simulink model "xEMU_SimulationModel3_rule1"  (R2017b)
settings: Solver=ode4  StartTime=0.0  StopTime=8192  FixedStep=0.01  RelTol=1e-3
undefined symbols (not defined in the file): a1, a2, a3, a4, ACO, BAT, Battery, DCT, DRT, EMS, ENV, Fahrzyklus_VS_modell, height_BAT, leistung, lib_bat, Maximum, Maximum_position, Num_cells, P_FC_max_long, P_FC_min_long, P_FC_step_max, Pbat_charge_max, Pbat_discharge_max, Pfc_max, Pfc_min, SOC_tar, time_peaks, TRM, velocity_peaks
libraries: simulink x5
(part 2 of 15)

== system xEMU_SimulationModel3_rule1/Fuel Cell System (FCS)/FC_controller  ==
  p_demand_ext : Inport
  V_dcLink : Inport  Port=2
  FC_state_BUS : Inport  Port=3
  V_FCS : Inport  Port=4
  p_fc_act : Inport  Port=5
  Add : Sum
  Bus Creator : BusCreator  Inputs=3
  Bus Creator1 : BusCreator  Inputs=5
  Constant : Constant  Value=42
  Constant1 : Constant  Value=P_FC_max_long
  Constant2 : Constant  Value=P_FC_step_max
  Constant4 : Constant  Value=P_FC_min_long
  Max : MinMax  Function=max  Inputs=2
  Min : MinMax  Inputs=2
  Product1 : Product  Inputs=*/
  Subtract : Sum  Inputs=+-
  Terminator : Terminator
  FCS_BUS : Outport
  i_demand : Outport  Port=2
  wires:
  Bus Creator1/1 -> Bus Creator/1
  FC_state_BUS/1 -> Bus Creator/2
  Constant/1 -> Bus Creator/3  "FCS_state"
  Add/1 -> Min/1
  Max/1 -> Bus Creator1/4  "P_FC_min"
  Min/1 -> Bus Creator1/2  "P_FC_max"
  Subtract/1 -> Max/1
  p_fc_act/1 -> Add/1, Subtract/1, Bus Creator1/1  "P_fc"
  Constant2/1 -> Add/2, Subtract/2
  Bus Creator/1 -> FCS_BUS/1
  V_dcLink/1 -> Terminator/1
  V_FCS/1 -> Product1/2
  Product1/1 -> i_demand/1
  Constant1/1 -> Min/2, Bus Creator1/3  "P_FC_max_long"
  Constant4/1 -> Max/2, Bus Creator1/5  "P_FC_min_long"
  p_demand_ext/1 -> Product1/1

== system xEMU_SimulationModel3_rule1/Fuel Cell System (FCS)/FC_system ==
  "P_fc " : Inport
  i_demand_dcdc_fc : Inport  Port=2
  1-D Lookup Table : Lookup_n-D  NumberOfTableDimensions=1  BreakpointsForDimension1=[0 10 20 50 126 241 270]  Table=[583 567 551 525 490 456 450]  InternalRulePriority=Speed  RndMeth=Simplest  InputSameDT=on
  Bus Creator : BusCreator  Inputs=2
  FaradayConstant : Constant  Commented=on  Value=96485
  FaradayConstant1 : Constant  Value=100
  MATLAB Function : MATLAB Function  TreatAsAtomicUnit=on
  NumCells : Constant  Commented=on  Value=Num_cells
  Product1 : Product  Commented=on  Inputs=/**
  Saturation : Saturate  UpperLimit=250  LowerLimit=0
  Scope : Scope
  Scope1 : Scope
  FCS_state_BUS : Outport
  V_FCS : Outport  Port=2
  i_act_fcs : Outport  Port=3
  wires:
  FaradayConstant1/1 -> Bus Creator/1  "H2_tankMass_kg"
  NumCells/1 -> Product1/3
  FaradayConstant/1 -> Product1/1
  Bus Creator/1 -> FCS_state_BUS/1
  1-D Lookup Table/1 -> Scope/1, V_FCS/1
  Saturation/1 -> Product1/2, i_act_fcs/1, 1-D Lookup Table/1
  i_demand_dcdc_fc/1 -> Scope1/1, Saturation/1
  MATLAB Function/1(H2_consumption_gramspersec) -> Bus Creator/2
  "P_fc "/1 -> MATLAB Function/1(xx)

== system xEMU_SimulationModel3_rule1/Scopes/Battery Scope ==
  Bus Selector : BusSelector  OutputSignals=V_bat,SOC,P_bat,I_bat
  Scope : Scope  NumInputPorts=3
  Scope1 : Scope
  Scope2 : Scope
  Scope6 : Scope
  wires:
  Bus Selector/1 -> Scope/1  "<V_bat>"
  [BAT_BUS] -> Bus Selector/1
  Bus Selector/2 -> Scope6/1  "<SOC>"
  [T_CellElement1] -> Scope1/1
  Bus Selector/3 -> Scope/3  "<P_bat>"
  Bus Selector/4 -> Scope2/1  "<I_bat>"

== system xEMU_SimulationModel3_rule1/Scopes/Energy Manager Scope ==
  Bus Selector1 : BusSelector  OutputSignals=P_acdc_Verlust,P_motor_mechanisch,P_motor_Verlust
  Bus Selector2 : BusSelector  OutputSignals=P_Klima
  Bus Selector3 : BusSelector  OutputSignals=P_bat
  Bus Selector4 : BusSelector  OutputSignals=signal1.P_fc
  Bus Selector5 : BusSelector  OutputSignals=P_dcdc_Verlust,P_dcLinkTractionLoad
  Divide : Product  Inputs=*/
  Integrator : Integrator
  Integrator1 : Integrator
  Leistung : Scope
  Leistung1 : Scope
  Leistung_verteilung : Scope
  Mux : Mux  Inputs=6
  Mux1 : Mux  Inputs=3
  wires:
  [DRT_BUS] -> Bus Selector1/1
  [DCT_BUS] -> Bus Selector5/1
  Mux/1 -> Leistung/1
  Bus Selector1/1 -> Mux/2  "<P_acdc_Verlust>"
  Bus Selector5/1 -> Integrator/1, Mux/5  "<P_dcdc_Verlust>"
  Bus Selector1/2 -> Mux/3  "<P_motor_mechanisch>"
  Bus Selector1/3 -> Mux/4  "<P_motor_Verlust>"
  [ACO_BUS] -> Bus Selector2/1
  Bus Selector2/1 -> Mux/6  "<P_Klima>"
  [APU_BUS] -> Mux/1
  [BAT_BUS] -> Bus Selector3/1
  Bus Selector3/1 -> Mux1/2  "<P_bat>"
  [FCS_BUS] -> Bus Selector4/1
  Bus Selector4/1 -> Mux1/3  "<P_fc>"
  Bus Selector5/2 -> Integrator1/1, Mux1/1  "<P_dcLinkTractionLoad>"
  Mux1/1 -> Leistung_verteilung/1
  Integrator/1 -> Divide/1
  Integrator1/1 -> Divide/2
  Divide/1 -> Leistung1/1

== system xEMU_SimulationModel3_rule1/Scopes/Fuel cell Scope  ==
  Bus Selector4 : BusSelector  OutputSignals=signal2.H2_tankMass_kg,signal2.H2_consumption_gramspersec
  Integrator : Integrator
  Scope : Scope  NumInputPorts=3
  wires:
  [FCS_BUS] -> Bus Selector4/1
  Bus Selector4/2 -> Scope/2, Integrator/1  "<H2_consumption_gramspersec>"
  Integrator/1 -> Scope/3  "Gesamtverbrauch_g"

== system xEMU_SimulationModel3_rule1/Scopes/Train Dynamics&Environment Scope ==
  Bus Selector1 : BusSelector  OutputSignals=v_drivingCycle_m/s,Steigung%
  Bus Selector2 : BusSelector  OutputSignals=v_train_m/s
  Integrator1 : Integrator
  Mux : Mux  Inputs=2
  Scope : Scope
  Scope2 : Scope
  V : Scope
  tag scope: distance=global
  wires:
  Bus Selector2/1 -> Mux/1  "<v_train_m/s>"
  [TRM_BUS] -> Bus Selector2/1
  [ENV_BUS] -> Bus Selector1/1
  Bus Selector1/1 -> Integrator1/1, Mux/2  "<v_drivingCycle_m/s>"
  Mux/1 -> V/1  "V_soll_VS_V_ist"
  Bus Selector1/2 -> Scope/1  "<Steigung%>"
  Integrator1/1 -> [distance], Scope2/1  "total distance"

== system xEMU_SimulationModel3_rule1/Train Dynamics (TRM)/Variant Subsystem ==
  v_drivingCycle_m/s : Inport
  h_drivingCycle_m : Inport  Port=2
  n_passengers_abs : Inport  Port=3
  adhesionCoefficient_abs : Inport  Port=4
  F_traction_N : Inport  Port=5
  v_s_model : Subsystem  VariantControl=Variant1
  v_t_model : Subsystem  VariantControl=Variant
  TRM_BUS : Outport
  F_tractionDemand_N : Outport  Port=2
  v_train_m/s : Outport  Port=3
  adhesionCoefficient : Outport  Port=4
  total_mass_kg : Outport  Port=5
  v_soll : Outport  Port=6

== system xEMU_SimulationModel3_rule1/Battery (BAT)_komplex/Subsystem/ActiveBalancing ==
  CellCurrents : Inport
  Demux : Demux  Outputs=1
  tag scope: ActBal1=global, BalancerBus=global
  wires:
  CellCurrents/1 -> Demux/1, [BalancerBus]
  Demux/1 -> [ActBal1]

== system xEMU_SimulationModel3_rule1/Battery (BAT)_komplex/Subsystem/CellCurrentMatrices ==
  Component0 : Subsystem
  Component1 : Subsystem
  Mux : Mux  Inputs=2
  Components : Outport
  wires:
  Mux/1 -> Components/1
  Component0/3(Value) -> Mux/1
  Component1/3(Value) -> Mux/2

== system xEMU_SimulationModel3_rule1/Battery (BAT)_komplex/Subsystem/CellCurrents ==
  CellCurrents : Inport
  Demux : Demux  Outputs=2
  Terminator : Terminator
  tag scope: I_CellElement1=global
  wires:
  CellCurrents/1 -> Demux/1
  Demux/2 -> Terminator/1
  Demux/1 -> [I_CellElement1]

== system xEMU_SimulationModel3_rule1/Battery (BAT)_komplex/Subsystem/CellPowerValues ==
  CellPower : Inport
  Demux : Demux  Outputs=1
  Out1 : Outport
  tag scope: P_CellElement1=global
  wires:
  CellPower/1 -> Out1/1, Demux/1  "CellPower"
  Demux/1 -> [P_CellElement1]

== system xEMU_SimulationModel3_rule1/Battery (BAT)_komplex/Subsystem/CellVoltageMatrices ==
  Component0 : Subsystem
  Component1 : Subsystem
  Mux : Mux  Inputs=2
  Components : Outport
  wires:
  Mux/1 -> Components/1
  Component0/3(Value) -> Mux/1
  Component1/3(Value) -> Mux/2

== system xEMU_SimulationModel3_rule1/Battery (BAT)_komplex/Subsystem/ElectricalCircuit ==
  Cellelement_Elem1 : Subsystem
  Out1 : Outport
  wires:
  Cellelement_Elem1/1(Out1) -> Out1/1

== system xEMU_SimulationModel3_rule1/Battery (BAT)_komplex/Subsystem/MatrixAxC ==
  StateComponent0 : Subsystem
  StateComponent1 : Subsystem
  StateComponent10 : Subsystem
  StateComponent11 : Subsystem
  StateComponent12 : Subsystem
  StateComponent13 : Subsystem
  StateComponent14 : Subsystem
  StateComponent15 : Subsystem
  StateComponent16 : Subsystem
  StateComponent17 : Subsystem
  StateComponent18 : Subsystem
  StateComponent2 : Subsystem
  StateComponent3 : Subsystem
  StateComponent4 : Subsystem
  StateComponent5 : Subsystem
  StateComponent6 : Subsystem
  StateComponent7 : Subsystem
  StateComponent8 : Subsystem
  StateComponent9 : Subsystem
  Components : Outport

== system xEMU_SimulationModel3_rule1/Battery (BAT)_komplex/Subsystem/MatrixX_alg ==
  Components : Outport

== system xEMU_SimulationModel3_rule1/Battery (BAT)_komplex/Subsystem/PowerMatrix ==
  Component0 : Subsystem
  Mux : Mux  Inputs=1
  Components : Outport
  wires:
  Mux/1 -> Components/1
  Component0/3(Value) -> Mux/1

== system xEMU_SimulationModel3_rule1/Battery (BAT)_komplex/Subsystem/SystemStates ==
  Mux : Mux  Inputs=19
  tag scope: StatesBus=global
  wires:
  [State1] -> Mux/1
  [State2] -> Mux/2
  [State3] -> Mux/3
  [State4] -> Mux/4
  [State5] -> Mux/5
  [State6] -> Mux/6
  [State7] -> Mux/7
  [State8] -> Mux/8
  [State9] -> Mux/9
  [State10] -> Mux/10
  [State11] -> Mux/11
  [State12] -> Mux/12
  [State13] -> Mux/13
  [State14] -> Mux/14
  [State15] -> Mux/15
  [State16] -> Mux/16
  [State17] -> Mux/17
  [State18] -> Mux/18
  [State19] -> Mux/19
  Mux/1 -> [StatesBus]

== system xEMU_SimulationModel3_rule1/Battery (BAT)_komplex/Subsystem/Thermal ==
  CellToFV : Subsystem
  ConductivityMatrix : MATLAB Function  TreatAsAtomicUnit=on
  Coolings : Subsystem
  FV Temperatures : Integrator  InitialCondition=[25.7297;25.7297;25.7297;25.7297;25.7297;25.7297;25.7297;25.7297;25.7297;25.7297;25.7297;25.7297;25.7297;25.7297;25.7297;25.7297;25.7297;25.7297;25.7297;25.7297;25.7297;25.7297;25.7297;25.7297;25.7297;25.7297;25.7297;25.7297;25.7297;25.7297;25.7297;25.7297;25.7297;25.7297;25.7297;25.7297;25.7297;25.7297;25.7297;25.7297;25.7297;25.7297;25.7297;25.7297;25.7297;25.7297;25.7297;25.7297;25.7297;25.7297;25.7297;25.7297;25.7297;25.7297;25.7297;25.7297;25.7297;25.7297;25.7297;25.7297;25.7297;25.7297;25.7297;25.7297;25.7297;25.7297;25.7297;25.7297;25.7297;25.7297;25.7297;25.7297;25.7297;25.7297;25.7297;25.7297;25.7297;25.7297;25.7297;25.7297;25.7297;25.7297;25.7297;25.7297;25.7297;25.7297;25.7297;25.7297;25.7297;25.7297;25.7297;25.7297;25.7297;25.7297;25.7297;25.7297;25.7297;25.7297;25.7297;25.7297;25.7297;25.7297;25.7297;25.7297;25.7297;25.7297;25.7297;25.7297;25.7297;25.7297;25.7297;25.7297;25.7297;25.7297;25.7297;25.7297;25.7297;25.7297;25.7297;25.7297;25.7297;25.7297;25.7297;25.7297;25.7297;25.7297;25.7297;25.7297;25.7297;25.7297;25.7297;25.7297;25.7297;25.7297;25.7297;25.7297;25.7297;25.7297;25.7297;25.7297;25.7297;25.7297;25.7297;25.7297;25.7297;25.7297;25.7297;25.7297;25.7297;25.7297;25.7297;25.7297;25.7297;25.7297;25.7297;25.7297;25.7297;25.7297;25.7297;25.7297;25.7297;25.7297;25.7297;25.7297;25.7297;25.7297;25.7297;25.7297;25.7297;25.7297;25.7297;25.7297;25.7297;25.7297;25.7297;25.7297;25.7297;25.7297;25.7297;25.7297;25.7297;25.7297;25.7297;25.7297;25.7297;25.7297;25.7297;25.7297;25.7297;25.7297;25.7297;25.7297;25.7297;25.7297;25.7297;25.7297;25.7297;25.7297;25.7297;25.7297;25.7297;25.7297;25.7297;25.7297;25.7297;25.7297;25.7297;25.7297;25.7297;25.7297;25.7297;25.7297;25.7297;25.7297;25.7297;25.7297;25.7297;25.7297;25.7297;25.7297;25.7297;25.7297;25.7297;25.7297;25.7297;25.7297;25.7297;25.7297;25.7297;25.7297;25.7297;25.7297;25.7297;25.7297;25.7297;25.7297;25.7297;25.7297;25.7297;25.7297;25.7297;25.7297;25.7297;25.7297;25.7297;25.7297;25.7297;25.7297;25.7297;25.7297;25.7297;25.7297;25.7297;25.7297;25.7297;25.7297;25.7297;25.7297;25.7297;25.7297;25.7297;25.7297;25.7297;25.7297;25.7297;25.7297;25.7297;25.7297;25.7297;25.7297;25.7297;25.7297;25.7297;25.7297;25.7297;25.7297;25.7297;25.7297;25.7297;25.7297;25.7297;25.7297;25.7297;25.7297;25.7297;25.7297;25.7297;25.7297;25.7297;25.7297;25.7297;25.7297;25.7297;25.7297;25.7297;25.7297;25.7297;25.7297;25.7297;25.7297]
  FVToCell : Subsystem
  Reciprocals of Thermal Capacities : Gain  Gain=[0.582768314846317;0.582768314846317;0.582768314846317;0.582768314846317;0.582768314846317;0.582768314846317;0.582768314846317;0.582768314846317;0.582768314846317;0.582768314846317;0.582768314846317;0.582768314846317;0.582768314846317;0.582768314846317;0.582768314846317;0.582768314846317;0.582768314846317;0.582768314846317;0.582768314846317;0.582768314846317;0.582768314846317;0.582768314846317;0.582768314846317;0.582768314846317;0.582768314846317;0.582768314846317;0.582768314846317;0.582768314846317;0.582768314846317;0.582768314846317;0.582768314846317;0.582768314846317;0.582768314846317;0.582768314846317;0.582768314846317;0.582768314846317;0.582768314846317;0.582768314846317;0.582768314846317;0.582768314846317;0.582768314846317;0.582768314846317;0.582768314846317;0.582768314846317;0.582768314846317;0.582768314846317;0.582768314846317;0.582768314846317;0.582768314846317;0.582768314846317;0.582768314846317;0.582768314846317;0.582768314846317;0.582768314846317;0.582768314846317;0.582768314846317;0.582768314846317;0.582768314846317;0.582768314846317;0.582768314846317;0.582768314846317;0.582768314846317;0.582768314846317;0.582768314846317;0.582768314846317;0.582768314846317;0.582768314846317;0.582768314846317;0.582768314846317;0.582768314846317;0.582768314846317;0.582768314846317;0.582768314846317;0.582768314846317;0.582768314846317;0.582768314846317;0.582768314846317;0.582768314846317;0.582768314846317;0.582768314846317;0.582768314846317;0.582768314846317;0.582768314846317;0.582768314846317;0.582768314846317;0.582768314846317;0.582768314846317;0.582768314846317;0.582768314846317;0.582768314846317;0.582768314846317;0.582768314846317;0.582768314846317;0.582768314846317;0.582768314846317;0.582768314846317;0.582768314846317;0.582768314846317;0.582768314846317;0.582768314846317;0.582768314846317;0.582768314846317;0.582768314846317;0.582768314846317;0.582768314846317;0.582768314846317;0.582768314846317;0.582768314846317;0.582768314846317;0.582768314846317;0.582768314846317;0.582768314846317;0.582768314846317;0.582768314846317;0.582768314846317;0.582768314846317;0.582768314846317;0.582768314846317;0.582768314846317;0.582768314846317;0.582768314846317;0.582768314846317;0.582768314846317;0.582768314846317;0.582768314846317;0.582768314846317;0.582768314846317;0.582768314846317;0.582768314846317;0.582768314846317;0.582768314846317;0.582768314846317;0.582768314846317;0.582768314846317;0.582768314846317;0.582768314846317;0.582768314846317;0.582768314846317;0.582768314846317;0.582768314846317;0.582768314846317;0.582768314846317;0.582768314846317;0.582768314846317;0.582768314846317;0.582768314846317;0.582768314846317;0.582768314846317;0.582768314846317;0.582768314846317;0.582768314846317;0.582768314846317;0.582768314846317;0.582768314846317;0.582768314846317;0.582768314846317;0.582768314846317;0.582768314846317;0.582768314846317;0.582768314846317;0.582768314846317;0.582768314846317;0.582768314846317;0.582768314846317;0.582768314846317;0.582768314846317;0.582768314846317;0.582768314846317;0.582768314846317;0.582768314846317;0.582768314846317;0.582768314846317;0.582768314846317;0.582768314846317;0.582768314846317;0.582768314846317;0.582768314846317;0.582768314846317;0.582768314846317;0.582768314846317;0.582768314846317;0.582768314846317;0.582768314846317;0.582768314846317;0.582768314846317;0.582768314846317;0.582768314846317;0.582768314846317;0.582768314846317;0.582768314846317;0.582768314846317;0.582768314846317;0.582768314846317;0.582768314846317;0.582768314846317;0.582768314846317;0.582768314846317;0.582768314846317;0.582768314846317;0.582768314846317;0.582768314846317;0.582768314846317;0.582768314846317;0.582768314846317;0.582768314846317;0.582768314846317;0.582768314846317;0.582768314846317;0.582768314846317;0.582768314846317;0.582768314846317;0.582768314846317;0.582768314846317;0.582768314846317;0.582768314846317;0.582768314846317;0.582768314846317;0.582768314846317;0.582768314846317;0.582768314846317;0.582768314846317;0.582768314846317 ...(+1404 chars)]
  Sum : Sum  Inputs=|+-+
  Out1 : Outport
  wires:
  ConductivityMatrix/1(y) -> Sum/3
  CellToFV/1(P_FV) -> Sum/1
  Coolings/1(P_FV) -> Sum/2
  FV Temperatures/1 -> FVToCell/1(T_FV), Coolings/1(T_FV), ConductivityMatrix/1(u)  "Temperatures"
  Reciprocals of Thermal Capacities/1 -> FV Temperatures/1
  Sum/1 -> Reciprocals of Thermal Capacities/1
  FVToCell/1(Out1) -> Out1/1

== system xEMU_SimulationModel3_rule1/Battery (BAT)_mittel/Battery/ActiveBalancing ==
  CellCurrents : Inport
  Demux : Demux  Outputs=1
  tag scope: ActBal1=scoped, BalancerBus=scoped
  wires:
  CellCurrents/1 -> Demux/1, [BalancerBus]
  Demux/1 -> [ActBal1]

== system xEMU_SimulationModel3_rule1/Battery (BAT)_mittel/Battery/CellCurrentMatrices ==
  Component0 : Subsystem
  Component1 : Subsystem
  Mux : Mux  Inputs=2
  Components : Outport
  wires:
  Mux/1 -> Components/1
  Component0/3(Value) -> Mux/1
  Component1/3(Value) -> Mux/2

== system xEMU_SimulationModel3_rule1/Battery (BAT)_mittel/Battery/CellCurrents ==
  CellCurrents : Inport
  Demux : Demux  Outputs=2
  Terminator : Terminator
  tag scope: I_CellElement1=scoped
  wires:
  CellCurrents/1 -> Demux/1
  Demux/2 -> Terminator/1
  Demux/1 -> [I_CellElement1]

== system xEMU_SimulationModel3_rule1/Battery (BAT)_mittel/Battery/CellPowerValues ==
  CellPower : Inport
  Demux : Demux  Outputs=1
  Out1 : Outport
  tag scope: P_CellElement1=scoped
  wires:
  CellPower/1 -> Demux/1, Out1/1
  Demux/1 -> [P_CellElement1]

== system xEMU_SimulationModel3_rule1/Battery (BAT)_mittel/Battery/CellVoltageMatrices ==
  Component0 : Subsystem
  Component1 : Subsystem
  Mux : Mux  Inputs=2
  Scope : Scope
  To Workspace : ToWorkspace  VariableName=Batt_volt_1s1p_thevenin  SaveFormat=Structure With Time  SampleTime=-1
  Components : Outport
  wires:
  Mux/1 -> Components/1
  Component0/3(Value) -> Mux/1
  Component1/3(Value) -> Scope/1, To Workspace/1, Mux/2

== system xEMU_SimulationModel3_rule1/Battery (BAT)_mittel/Battery/ElectricalCircuit ==
  GotoTag1 : GotoTagVisibility  GotoTag=SoC1
  SerialTwoPort_Elem1 : Subsystem
  SoC_Bus : BusCreator  Inputs=1
  SoC_%_Bus : Outport
  wires:
  [SoC1] -> SoC_Bus/1
  SoC_Bus/1 -> SoC_%_Bus/1

== system xEMU_SimulationModel3_rule1/Battery (BAT)_mittel/Battery/MatrixAxC ==
  StateComponent0 : Subsystem
  StateComponent1 : Subsystem
  StateComponent2 : Subsystem
  Components : Outport

== system xEMU_SimulationModel3_rule1/Battery (BAT)_mittel/Battery/MatrixX_alg ==
  Components : Outport

== system xEMU_SimulationModel3_rule1/Battery (BAT)_mittel/Battery/PowerMatrix ==
  Component0 : Subsystem
  Mux : Mux  Inputs=1
  Components : Outport
  wires:
  Mux/1 -> Components/1
  Component0/3(Value) -> Mux/1

== system xEMU_SimulationModel3_rule1/Battery (BAT)_mittel/Battery/SystemStates ==
  Mux : Mux  Inputs=3
  tag scope: StatesBus=scoped
  wires:
  [State1] -> Mux/1
  [State2] -> Mux/2
  [State3] -> Mux/3
  Mux/1 -> [StatesBus]

== system xEMU_SimulationModel3_rule1/Battery (BAT)_mittel/Battery/Thermal ==
  CellTempBus : BusCreator  Inputs=1
  CellToFV : Subsystem
  ConductivityMatrix : MATLAB Function  TreatAsAtomicUnit=on
  Coolings : Subsystem
  FV Temperatures : Integrator  InitialCondition=[25.7297;25.7297;25.7297;25.7297;25.7297;25.7297;25.7297;25.7297;25.7297;25.7297;25.7297;25.7297;25.7297;25.7297;25.7297;25.7297;25.7297;25.7297;25.7297;25.7297;25.7297;25.7297;25.7297;25.7297;25.7297;25.7297;25.7297;25.7297;25.7297;25.7297;25.7297;25.7297;25.7297;25.7297;25.7297;25.7297;25.7297;25.7297;25.7297;25.7297;25.7297;25.7297;25.7297;25.7297;25.7297;25.7297;25.7297;25.7297;25.7297;25.7297;25.7297;25.7297;25.7297;25.7297;25.7297;25.7297;25.7297;25.7297;25.7297;25.7297;25.7297;25.7297;25.7297;25.7297;25.7297;25.7297;25.7297;25.7297;25.7297;25.7297;25.7297;25.7297;25.7297;25.7297;25.7297;25.7297;25.7297;25.7297;25.7297;25.7297;25.7297;25.7297;25.7297;25.7297;25.7297;25.7297;25.7297;25.7297;25.7297;25.7297;25.7297;25.7297;25.7297;25.7297;25.7297;25.7297;25.7297;25.7297;25.7297;25.7297;25.7297;25.7297;25.7297;25.7297;25.7297;25.7297;25.7297;25.7297;25.7297;25.7297;25.7297;25.7297;25.7297;25.7297;25.7297;25.7297;25.7297;25.7297;25.7297;25.7297;25.7297;25.7297;25.7297;25.7297;25.7297;25.7297;25.7297;25.7297;25.7297;25.7297;25.7297;25.7297;25.7297;25.7297;25.7297;25.7297;25.7297;25.7297;25.7297;25.7297;25.7297;25.7297;25.7297;25.7297;25.7297;25.7297;25.7297;25.7297;25.7297;25.7297;25.7297;25.7297;25.7297;25.7297;25.7297;25.7297;25.7297;25.7297;25.7297;25.7297;25.7297;25.7297;25.7297;25.7297;25.7297;25.7297;25.7297;25.7297;25.7297;25.7297;25.7297;25.7297;25.7297;25.7297;25.7297;25.7297;25.7297;25.7297;25.7297;25.7297;25.7297;25.7297;25.7297;25.7297;25.7297;25.7297;25.7297;25.7297;25.7297;25.7297;25.7297;25.7297;25.7297;25.7297;25.7297;25.7297;25.7297;25.7297;25.7297;25.7297;25.7297;25.7297;25.7297;25.7297;25.7297;25.7297;25.7297;25.7297;25.7297;25.7297;25.7297;25.7297;25.7297;25.7297;25.7297;25.7297;25.7297;25.7297;25.7297;25.7297;25.7297;25.7297;25.7297;25.7297;25.7297;25.7297;25.7297;25.7297;25.7297;25.7297;25.7297;25.7297;25.7297;25.7297;25.7297;25.7297;25.7297;25.7297;25.7297;25.7297;25.7297;25.7297;25.7297;25.7297;25.7297;25.7297;25.7297;25.7297;25.7297;25.7297;25.7297;25.7297;25.7297;25.7297;25.7297;25.7297;25.7297;25.7297;25.7297;25.7297;25.7297;25.7297;25.7297;25.7297;25.7297;25.7297;25.7297;25.7297;25.7297;25.7297;25.7297;25.7297;25.7297;25.7297;25.7297;25.7297;25.7297;25.7297;25.7297;25.7297;25.7297;25.7297;25.7297;25.7297;25.7297;25.7297;25.7297;25.7297;25.7297;25.7297;25.7297;25.7297;25.7297;25.7297;25.7297;25.7297;25.7297;25.7297;25.7297;25.7297]
  FVToCell : Subsystem
  Reciprocals of Thermal Capacities : Gain  Gain=[0.582768314846317;0.582768314846317;0.582768314846317;0.582768314846317;0.582768314846317;0.582768314846317;0.582768314846317;0.582768314846317;0.582768314846317;0.582768314846317;0.582768314846317;0.582768314846317;0.582768314846317;0.582768314846317;0.582768314846317;0.582768314846317;0.582768314846317;0.582768314846317;0.582768314846317;0.582768314846317;0.582768314846317;0.582768314846317;0.582768314846317;0.582768314846317;0.582768314846317;0.582768314846317;0.582768314846317;0.582768314846317;0.582768314846317;0.582768314846317;0.582768314846317;0.582768314846317;0.582768314846317;0.582768314846317;0.582768314846317;0.582768314846317;0.582768314846317;0.582768314846317;0.582768314846317;0.582768314846317;0.582768314846317;0.582768314846317;0.582768314846317;0.582768314846317;0.582768314846317;0.582768314846317;0.582768314846317;0.582768314846317;0.582768314846317;0.582768314846317;0.582768314846317;0.582768314846317;0.582768314846317;0.582768314846317;0.582768314846317;0.582768314846317;0.582768314846317;0.582768314846317;0.582768314846317;0.582768314846317;0.582768314846317;0.582768314846317;0.582768314846317;0.582768314846317;0.582768314846317;0.582768314846317;0.582768314846317;0.582768314846317;0.582768314846317;0.582768314846317;0.582768314846317;0.582768314846317;0.582768314846317;0.582768314846317;0.582768314846317;0.582768314846317;0.582768314846317;0.582768314846317;0.582768314846317;0.582768314846317;0.582768314846317;0.582768314846317;0.582768314846317;0.582768314846317;0.582768314846317;0.582768314846317;0.582768314846317;0.582768314846317;0.582768314846317;0.582768314846317;0.582768314846317;0.582768314846317;0.582768314846317;0.582768314846317;0.582768314846317;0.582768314846317;0.582768314846317;0.582768314846317;0.582768314846317;0.582768314846317;0.582768314846317;0.582768314846317;0.582768314846317;0.582768314846317;0.582768314846317;0.582768314846317;0.582768314846317;0.582768314846317;0.582768314846317;0.582768314846317;0.582768314846317;0.582768314846317;0.582768314846317;0.582768314846317;0.582768314846317;0.582768314846317;0.582768314846317;0.582768314846317;0.582768314846317;0.582768314846317;0.582768314846317;0.582768314846317;0.582768314846317;0.582768314846317;0.582768314846317;0.582768314846317;0.582768314846317;0.582768314846317;0.582768314846317;0.582768314846317;0.582768314846317;0.582768314846317;0.582768314846317;0.582768314846317;0.582768314846317;0.582768314846317;0.582768314846317;0.582768314846317;0.582768314846317;0.582768314846317;0.582768314846317;0.582768314846317;0.582768314846317;0.582768314846317;0.582768314846317;0.582768314846317;0.582768314846317;0.582768314846317;0.582768314846317;0.582768314846317;0.582768314846317;0.582768314846317;0.582768314846317;0.582768314846317;0.582768314846317;0.582768314846317;0.582768314846317;0.582768314846317;0.582768314846317;0.582768314846317;0.582768314846317;0.582768314846317;0.582768314846317;0.582768314846317;0.582768314846317;0.582768314846317;0.582768314846317;0.582768314846317;0.582768314846317;0.582768314846317;0.582768314846317;0.582768314846317;0.582768314846317;0.582768314846317;0.582768314846317;0.582768314846317;0.582768314846317;0.582768314846317;0.582768314846317;0.582768314846317;0.582768314846317;0.582768314846317;0.582768314846317;0.582768314846317;0.582768314846317;0.582768314846317;0.582768314846317;0.582768314846317;0.582768314846317;0.582768314846317;0.582768314846317;0.582768314846317;0.582768314846317;0.582768314846317;0.582768314846317;0.582768314846317;0.582768314846317;0.582768314846317;0.582768314846317;0.582768314846317;0.582768314846317;0.582768314846317;0.582768314846317;0.582768314846317;0.582768314846317;0.582768314846317;0.582768314846317;0.582768314846317;0.582768314846317;0.582768314846317;0.582768314846317;0.582768314846317;0.582768314846317;0.582768314846317;0.582768314846317;0.582768314846317;0.582768314846317;0.582768314846317;0.582768314846317;0.582768314846317;0.582768314846317;0.582768314846317 ...(+1404 chars)]
  Scope : Scope
  Sum : Sum  Inputs=|+-+
  CellTemp_Bus : Outport
  wires:
  ConductivityMatrix/1(y) -> Sum/3
  CellToFV/1(P_FV) -> Sum/1
  Coolings/1(P_FV) -> Scope/1, Sum/2
  FV Temperatures/1 -> FVToCell/1(T_FV), Coolings/1(T_FV), ConductivityMatrix/1(u)  "Temperatures"
  Reciprocals of Thermal Capacities/1 -> FV Temperatures/1
  Sum/1 -> Reciprocals of Thermal Capacities/1
  FVToCell/1(Out1) -> CellTempBus/1
  CellTempBus/1 -> CellTemp_Bus/1

== system xEMU_SimulationModel3_rule1/Battery (BAT)_mittel/Subsystem1/ActiveBalancing ==
  CellCurrents : Inport
  Demux : Demux  Outputs=1
  tag scope: ActBal1=global, BalancerBus=global
  wires:
  CellCurrents/1 -> Demux/1, [BalancerBus]
  Demux/1 -> [ActBal1]

== system xEMU_SimulationModel3_rule1/Battery (BAT)_mittel/Subsystem1/CellCurrentMatrices ==
  Component0 : Subsystem
  Component1 : Subsystem
  Mux : Mux  Inputs=2
  Components : Outport
  wires:
  Mux/1 -> Components/1
  Component0/3(Value) -> Mux/1
  Component1/3(Value) -> Mux/2

== system xEMU_SimulationModel3_rule1/Battery (BAT)_mittel/Subsystem1/CellCurrents ==
  CellCurrents : Inport
  Demux : Demux  Outputs=2
  Terminator : Terminator
  tag scope: I_CellElement1=global
  wires:
  CellCurrents/1 -> Demux/1
  Demux/2 -> Terminator/1
  Demux/1 -> [I_CellElement1]

== system xEMU_SimulationModel3_rule1/Battery (BAT)_mittel/Subsystem1/CellPowerValues ==
  CellPower : Inport
  Demux : Demux  Outputs=1
  Out1 : Outport
  tag scope: P_CellElement1=global
  wires:
  CellPower/1 -> Out1/1, Demux/1  "CellPower"
  Demux/1 -> [P_CellElement1]

== system xEMU_SimulationModel3_rule1/Battery (BAT)_mittel/Subsystem1/CellVoltageMatrices ==
  Component0 : Subsystem
  Component1 : Subsystem
  Mux : Mux  Inputs=2
  Components : Outport
  wires:
  Mux/1 -> Components/1
  Component0/3(Value) -> Mux/1
  Component1/3(Value) -> Mux/2

== system xEMU_SimulationModel3_rule1/Battery (BAT)_mittel/Subsystem1/ElectricalCircuit ==
  Cellelement_Elem1 : Subsystem
  Out1 : Outport
  wires:
  Cellelement_Elem1/1(Out1) -> Out1/1

== system xEMU_SimulationModel3_rule1/Battery (BAT)_mittel/Subsystem1/MatrixAxC ==
  StateComponent0 : Subsystem
  StateComponent1 : Subsystem
  StateComponent10 : Subsystem
  StateComponent11 : Subsystem
  StateComponent12 : Subsystem
  StateComponent13 : Subsystem
  StateComponent14 : Subsystem
  StateComponent15 : Subsystem
  StateComponent16 : Subsystem
  StateComponent17 : Subsystem
  StateComponent18 : Subsystem
  StateComponent2 : Subsystem
  StateComponent3 : Subsystem
  StateComponent4 : Subsystem
  StateComponent5 : Subsystem
  StateComponent6 : Subsystem
  StateComponent7 : Subsystem
  StateComponent8 : Subsystem
  StateComponent9 : Subsystem
  Components : Outport

== system xEMU_SimulationModel3_rule1/Battery (BAT)_mittel/Subsystem1/MatrixX_alg ==
  Components : Outport

== system xEMU_SimulationModel3_rule1/Battery (BAT)_mittel/Subsystem1/PowerMatrix ==
  Component0 : Subsystem
  Mux : Mux  Inputs=1
  Components : Outport
  wires:
  Mux/1 -> Components/1
  Component0/3(Value) -> Mux/1

== system xEMU_SimulationModel3_rule1/Battery (BAT)_mittel/Subsystem1/SystemStates ==
  Mux : Mux  Inputs=19
  tag scope: StatesBus=global
  wires:
  [State1] -> Mux/1
  [State2] -> Mux/2
  [State3] -> Mux/3
  [State4] -> Mux/4
  [State5] -> Mux/5
  [State6] -> Mux/6
  [State7] -> Mux/7
  [State8] -> Mux/8
  [State9] -> Mux/9
  [State10] -> Mux/10
  [State11] -> Mux/11
  [State12] -> Mux/12
  [State13] -> Mux/13
  [State14] -> Mux/14
  [State15] -> Mux/15
  [State16] -> Mux/16
  [State17] -> Mux/17
  [State18] -> Mux/18
  [State19] -> Mux/19
  Mux/1 -> [StatesBus]

== system xEMU_SimulationModel3_rule1/Battery (BAT)_mittel/Subsystem1/Thermal ==
  CellToFV : Subsystem
  ConductivityMatrix : MATLAB Function  TreatAsAtomicUnit=on
  Coolings : Subsystem
  FV Temperatures : Integrator  InitialCondition=[25.7297;25.7297;25.7297;25.7297;25.7297;25.7297;25.7297;25.7297;25.7297;25.7297;25.7297;25.7297;25.7297;25.7297;25.7297;25.7297;25.7297;25.7297;25.7297;25.7297;25.7297;25.7297;25.7297;25.7297;25.7297;25.7297;25.7297;25.7297;25.7297;25.7297;25.7297;25.7297;25.7297;25.7297;25.7297;25.7297;25.7297;25.7297;25.7297;25.7297;25.7297;25.7297;25.7297;25.7297;25.7297;25.7297;25.7297;25.7297;25.7297;25.7297;25.7297;25.7297;25.7297;25.7297;25.7297;25.7297;25.7297;25.7297;25.7297;25.7297;25.7297;25.7297;25.7297;25.7297;25.7297;25.7297;25.7297;25.7297;25.7297;25.7297;25.7297;25.7297;25.7297;25.7297;25.7297;25.7297;25.7297;25.7297;25.7297;25.7297;25.7297;25.7297;25.7297;25.7297;25.7297;25.7297;25.7297;25.7297;25.7297;25.7297;25.7297;25.7297;25.7297;25.7297;25.7297;25.7297;25.7297;25.7297;25.7297;25.7297;25.7297;25.7297;25.7297;25.7297;25.7297;25.7297;25.7297;25.7297;25.7297;25.7297;25.7297;25.7297;25.7297;25.7297;25.7297;25.7297;25.7297;25.7297;25.7297;25.7297;25.7297;25.7297;25.7297;25.7297;25.7297;25.7297;25.7297;25.7297;25.7297;25.7297;25.7297;25.7297;25.7297;25.7297;25.7297;25.7297;25.7297;25.7297;25.7297;25.7297;25.7297;25.7297;25.7297;25.7297;25.7297;25.7297;25.7297;25.7297;25.7297;25.7297;25.7297;25.7297;25.7297;25.7297;25.7297;25.7297;25.7297;25.7297;25.7297;25.7297;25.7297;25.7297;25.7297;25.7297;25.7297;25.7297;25.7297;25.7297;25.7297;25.7297;25.7297;25.7297;25.7297;25.7297;25.7297;25.7297;25.7297;25.7297;25.7297;25.7297;25.7297;25.7297;25.7297;25.7297;25.7297;25.7297;25.7297;25.7297;25.7297;25.7297;25.7297;25.7297;25.7297;25.7297;25.7297;25.7297;25.7297;25.7297;25.7297;25.7297;25.7297;25.7297;25.7297;25.7297;25.7297;25.7297;25.7297;25.7297;25.7297;25.7297;25.7297;25.7297;25.7297;25.7297;25.7297;25.7297;25.7297;25.7297;25.7297;25.7297;25.7297;25.7297;25.7297;25.7297;25.7297;25.7297;25.7297;25.7297;25.7297;25.7297;25.7297;25.7297;25.7297;25.7297;25.7297;25.7297;25.7297;25.7297;25.7297;25.7297;25.7297;25.7297;25.7297;25.7297;25.7297;25.7297;25.7297;25.7297;25.7297;25.7297;25.7297;25.7297;25.7297;25.7297;25.7297;25.7297;25.7297;25.7297;25.7297;25.7297;25.7297;25.7297;25.7297;25.7297;25.7297;25.7297;25.7297;25.7297;25.7297;25.7297;25.7297;25.7297;25.7297;25.7297;25.7297;25.7297;25.7297;25.7297;25.7297;25.7297;25.7297;25.7297;25.7297;25.7297;25.7297;25.7297;25.7297;25.7297;25.7297;25.7297;25.7297;25.7297;25.7297;25.7297;25.7297;25.7297;25.7297;25.7297;25.7297;25.7297]
  FVToCell : Subsystem
  Reciprocals of Thermal Capacities : Gain  Gain=[0.582768314846317;0.582768314846317;0.582768314846317;0.582768314846317;0.582768314846317;0.582768314846317;0.582768314846317;0.582768314846317;0.582768314846317;0.582768314846317;0.582768314846317;0.582768314846317;0.582768314846317;0.582768314846317;0.582768314846317;0.582768314846317;0.582768314846317;0.582768314846317;0.582768314846317;0.582768314846317;0.582768314846317;0.582768314846317;0.582768314846317;0.582768314846317;0.582768314846317;0.582768314846317;0.582768314846317;0.582768314846317;0.582768314846317;0.582768314846317;0.582768314846317;0.582768314846317;0.582768314846317;0.582768314846317;0.582768314846317;0.582768314846317;0.582768314846317;0.582768314846317;0.582768314846317;0.582768314846317;0.582768314846317;0.582768314846317;0.582768314846317;0.582768314846317;0.582768314846317;0.582768314846317;0.582768314846317;0.582768314846317;0.582768314846317;0.582768314846317;0.582768314846317;0.582768314846317;0.582768314846317;0.582768314846317;0.582768314846317;0.582768314846317;0.582768314846317;0.582768314846317;0.582768314846317;0.582768314846317;0.582768314846317;0.582768314846317;0.582768314846317;0.582768314846317;0.582768314846317;0.582768314846317;0.582768314846317;0.582768314846317;0.582768314846317;0.582768314846317;0.582768314846317;0.582768314846317;0.582768314846317;0.582768314846317;0.582768314846317;0.582768314846317;0.582768314846317;0.582768314846317;0.582768314846317;0.582768314846317;0.582768314846317;0.582768314846317;0.582768314846317;0.582768314846317;0.582768314846317;0.582768314846317;0.582768314846317;0.582768314846317;0.582768314846317;0.582768314846317;0.582768314846317;0.582768314846317;0.582768314846317;0.582768314846317;0.582768314846317;0.582768314846317;0.582768314846317;0.582768314846317;0.582768314846317;0.582768314846317;0.582768314846317;0.582768314846317;0.582768314846317;0.582768314846317;0.582768314846317;0.582768314846317;0.582768314846317;0.582768314846317;0.582768314846317;0.582768314846317;0.582768314846317;0.582768314846317;0.582768314846317;0.582768314846317;0.582768314846317;0.582768314846317;0.582768314846317;0.582768314846317;0.582768314846317;0.582768314846317;0.582768314846317;0.582768314846317;0.582768314846317;0.582768314846317;0.582768314846317;0.582768314846317;0.582768314846317;0.582768314846317;0.582768314846317;0.582768314846317;0.582768314846317;0.582768314846317;0.582768314846317;0.582768314846317;0.582768314846317;0.582768314846317;0.582768314846317;0.582768314846317;0.582768314846317;0.582768314846317;0.582768314846317;0.582768314846317;0.582768314846317;0.582768314846317;0.582768314846317;0.582768314846317;0.582768314846317;0.582768314846317;0.582768314846317;0.582768314846317;0.582768314846317;0.582768314846317;0.582768314846317;0.582768314846317;0.582768314846317;0.582768314846317;0.582768314846317;0.582768314846317;0.582768314846317;0.582768314846317;0.582768314846317;0.582768314846317;0.582768314846317;0.582768314846317;0.582768314846317;0.582768314846317;0.582768314846317;0.582768314846317;0.582768314846317;0.582768314846317;0.582768314846317;0.582768314846317;0.582768314846317;0.582768314846317;0.582768314846317;0.582768314846317;0.582768314846317;0.582768314846317;0.582768314846317;0.582768314846317;0.582768314846317;0.582768314846317;0.582768314846317;0.582768314846317;0.582768314846317;0.582768314846317;0.582768314846317;0.582768314846317;0.582768314846317;0.582768314846317;0.582768314846317;0.582768314846317;0.582768314846317;0.582768314846317;0.582768314846317;0.582768314846317;0.582768314846317;0.582768314846317;0.582768314846317;0.582768314846317;0.582768314846317;0.582768314846317;0.582768314846317;0.582768314846317;0.582768314846317;0.582768314846317;0.582768314846317;0.582768314846317;0.582768314846317;0.582768314846317;0.582768314846317;0.582768314846317;0.582768314846317;0.582768314846317;0.582768314846317;0.582768314846317;0.582768314846317;0.582768314846317;0.582768314846317;0.582768314846317;0.582768314846317;0.582768314846317 ...(+1404 chars)]
  Sum : Sum  Inputs=|+-+
  Out1 : Outport
  wires:
  ConductivityMatrix/1(y) -> Sum/3
  CellToFV/1(P_FV) -> Sum/1
  Coolings/1(P_FV) -> Sum/2
  FV Temperatures/1 -> FVToCell/1(T_FV), Coolings/1(T_FV), ConductivityMatrix/1(u)  "Temperatures"
  Reciprocals of Thermal Capacities/1 -> FV Temperatures/1
  Sum/1 -> Reciprocals of Thermal Capacities/1
  FVToCell/1(Out1) -> Out1/1

== system xEMU_SimulationModel3_rule1/Battery (BAT)_mittel_02/Cell/ActiveBalancing ==
  CellCurrents : Inport
  Demux : Demux  Outputs=1
  tag scope: ActBal1=global, BalancerBus=global
  wires:
  CellCurrents/1 -> Demux/1, [BalancerBus]
  Demux/1 -> [ActBal1]

== system xEMU_SimulationModel3_rule1/Battery (BAT)_mittel_02/Cell/CellCurrentMatrices ==
  Component0 : Subsystem
  Mux : Mux  Inputs=1
  Components : Outport
  wires:
  Mux/1 -> Components/1
  Component0/3(Value) -> Mux/1

== system xEMU_SimulationModel3_rule1/Battery (BAT)_mittel_02/Cell/CellCurrents ==
  CellCurrents : Inport
  Demux : Demux  Outputs=1
  tag scope: I_CellElement1=global
  wires:
  CellCurrents/1 -> Demux/1
  Demux/1 -> [I_CellElement1]

== system xEMU_SimulationModel3_rule1/Battery (BAT)_mittel_02/Cell/CellPowerValues ==
  CellPower : Inport
  Demux : Demux  Outputs=1
  tag scope: P_CellElement1=global
  wires:
  CellPower/1 -> Demux/1
  Demux/1 -> [P_CellElement1]

== system xEMU_SimulationModel3_rule1/Battery (BAT)_mittel_02/Cell/CellVoltageMatrices ==
  Component0 : Subsystem
  Mux : Mux  Inputs=1
  Components : Outport
  wires:
  Mux/1 -> Components/1
  Component0/3(Value) -> Mux/1

== system xEMU_SimulationModel3_rule1/Battery (BAT)_mittel_02/Cell/ElectricalCircuit ==
  SerialTwoPort_Elem1 : Subsystem

== system xEMU_SimulationModel3_rule1/Battery (BAT)_mittel_02/Cell/MatrixAxC ==
  StateComponent0 : Subsystem
  StateComponent1 : Subsystem
  StateComponent2 : Subsystem
  Components : Outport

== system xEMU_SimulationModel3_rule1/Battery (BAT)_mittel_02/Cell/MatrixX_alg ==
  Components : Outport

== system xEMU_SimulationModel3_rule1/Battery (BAT)_mittel_02/Cell/PowerMatrix ==
  Component0 : Subsystem
  Mux : Mux  Inputs=1
  Components : Outport
  wires:
  Mux/1 -> Components/1
  Component0/3(Value) -> Mux/1

== system xEMU_SimulationModel3_rule1/Battery (BAT)_mittel_02/Cell/SoC_Vector ==
  Mux : Mux  Inputs=1
  SocVector : Outport
  wires:
  Mux/1 -> SocVector/1
  [SoC_CellElement1] -> Mux/1

== system xEMU_SimulationModel3_rule1/Battery (BAT)_mittel_02/Cell/SystemStates ==
  Mux : Mux  Inputs=3
  tag scope: StatesBus=global
  wires:
  [State1] -> Mux/1
  [State2] -> Mux/2
  [State3] -> Mux/3
  Mux/1 -> [StatesBus]

== system xEMU_SimulationModel3_rule1/Battery (BAT)_mittel_02/Cell/Temperature_Vector ==
  Mux : Mux  Inputs=1
  TemperatureVector : Outport
  wires:
  Mux/1 -> TemperatureVector/1
  [T_CellElement1] -> Mux/1
